simulink model "PassStFwdBkwdIsPosChk"  (R2018b)
settings: Solver=FixedStepDiscrete  StartTime=0.0  StopTime=10.0  RelTol=1e-3
undefined symbols (not defined in the file or in its folder): KeSMSuFirstRwStFwdBkwdPosDelta_Val, KeSMSuFirstRwStFwdBkwdPosTolr_Val
settings Model: Creator=sn2xws  LastModifiedBy=sn2xws
settings Model: ModifiedHistory=|
  | 2024.7.5 V3.0.0 557模式流程V1.9
  | 2024.8.14 V3.0.1 NotMovFlg从库函数中移出
settings DataIOCC: SaveFormat=StructureWithTime
settings OptimizationCC: DefaultParameterBehavior=Inlined  EnhancedBackFolding=on  PassReuseOutputArgsAs=Individual arguments  ZeroExternalMemoryAtStartup=off  ZeroInternalMemoryAtStartup=off  OptimizeBlockOrder=speed  DifferentSizesBufferReuse=on  OptimizationCustomize=off
settings DebuggingCC: ParameterTunabilityLossMsg=error
settings SFSimCC: MATLABDynamicMemAlloc=off
settings RTWCC: SystemTargetFile=autosar.tlc  GenCodeOnly=on  TemplateMakefile=ert_default_tmf  Description=AUTOSAR  GenerateReport=on  IncludeHyperlinkInReport=on  LaunchReport=on  GenerateTraceInfo=on  GenerateTraceReport=on  GenerateTraceReportSl=on  GenerateTraceReportSf=on  GenerateTraceReportEml=on
settings CodeAppCC: ForceParamTrailComments=on  IgnoreCustomStorageClasses=off  OperatorAnnotations=on  SimulinkDataObjDesc=on  SFDataObjDesc=on  InsertBlockDesc=on
settings STFCustomTargetCC: TargetLangStandard=C99 (ISO)  MultiwordLength=256  ParMdlRefBuildCompliant=on  CompOptLevelCompliant=on  IncludeMdlTerminateFcn=off  CombineOutputUpdateFcns=on  SuppressErrorStatus=on  ERTCustomFileBanners=on  SupportNonFinite=off  SupportComplex=off  SupportContinuousTime=off  SupportNonInlinedSFcns=off  RemoveResetFunc=on  MATLABClassNameForMDSCustomization=Simulink.SoftwareTarget.ERTCustomization  AutosarCompliant=on  UseToolchainInfoCompliant=on  LookupTableObjectStructAxisOrder=2,1,3,4,...  LUTObjectStructOrderEvenSpacing=Size,Table,Breakpoints  SystemTargetFile=autosar.tlc
settings ERTTargetCC: TargetLangStandard=C99 (ISO)  ConcurrentExecutionCompliant=off  IncludeMdlTerminateFcn=off  SuppressErrorStatus=on  SupportNonFinite=off  SupportComplex=off  ModelStepFunctionPrototypeControlCompliant=off  CPPClassGenCompliant=off  AutosarCompliant=on  LookupTableObjectStructAxisOrder=2,1,3,4,...  LUTObjectStructOrderEvenSpacing=Size,Table,Breakpoints  InlinedParameterPlacement=NonHierarchical  ERTCustomFileTemplate=example_file_process.tlc  ERTFilePackagingFormat=Compact

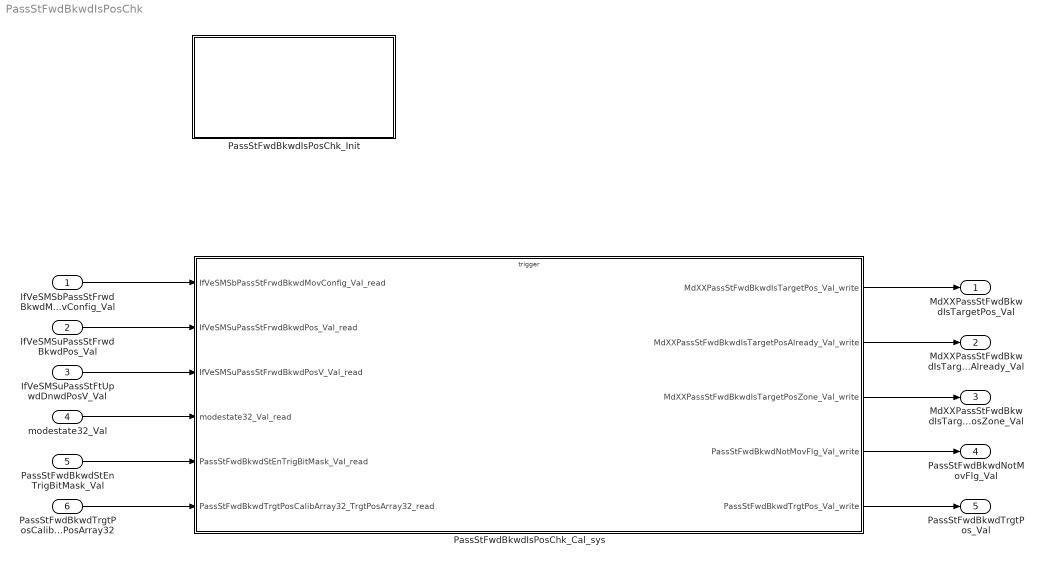
== system PassStFwdBkwdIsPosChk ==
  IfVeSMSbPassStFrwdBkwdMovConfig_Val : Inport  OutDataTypeStr=boolean  PortDimensions=1
  IfVeSMSuPassStFrwdBkwdPos_Val : Inport  Port=2  OutDataTypeStr=uint16  PortDimensions=1
  IfVeSMSuPassStFtUpwdDnwdPosV_Val : Inport  Port=3  OutDataTypeStr=boolean  PortDimensions=1
  modestate32_Val : Inport  Port=4  OutDataTypeStr=uint32  PortDimensions=1
  PassStFwdBkwdStEnTrigBitMask_Val : Inport  Port=5  OutDataTypeStr=uint32  PortDimensions=1
  PassStFwdBkwdTrgtPosCalibArray32_TrgtPosArray32 : Inport  Description=|  Port=6  OutDataTypeStr=uint16  PortDimensions=96
      | 0:Pos
      | 1:Max
      | 2:Min
  PassStFwdBkwdIsPosChk_Cal_sys : Subsystem
  PassStFwdBkwdIsPosChk_Init : Subsystem
  MdXXPassStFwdBkwdIsTargetPos_Val : Outport  OutDataTypeStr=uint32  PortDimensions=1
  MdXXPassStFwdBkwdIsTargetPosAlready_Val : Outport  Port=2  OutDataTypeStr=uint32  PortDimensions=1
  MdXXPassStFwdBkwdIsTargetPosZone_Val : Outport  Port=3  OutDataTypeStr=uint32  PortDimensions=1
  PassStFwdBkwdNotMovFlg_Val : Outport  Port=4  OutDataTypeStr=boolean  PortDimensions=1
  PassStFwdBkwdTrgtPos_Val : Outport  Port=5  OutDataTypeStr=uint16  PortDimensions=1
  wires:
  IfVeSMSbPassStFrwdBkwdMovConfig_Val/1 -> PassStFwdBkwdIsPosChk_Cal_sys/1(IfVeSMSbPassStFrwdBkwdMovConfig_Val_read)
  IfVeSMSuPassStFrwdBkwdPos_Val/1 -> PassStFwdBkwdIsPosChk_Cal_sys/2(IfVeSMSuPassStFrwdBkwdPos_Val_read)
  IfVeSMSuPassStFtUpwdDnwdPosV_Val/1 -> PassStFwdBkwdIsPosChk_Cal_sys/3(IfVeSMSuPassStFrwdBkwdPosV_Val_read)
  modestate32_Val/1 -> PassStFwdBkwdIsPosChk_Cal_sys/4(modestate32_Val_read)
  PassStFwdBkwdStEnTrigBitMask_Val/1 -> PassStFwdBkwdIsPosChk_Cal_sys/5(PassStFwdBkwdStEnTrigBitMask_Val_read)
  PassStFwdBkwdTrgtPosCalibArray32_TrgtPosArray32/1 -> PassStFwdBkwdIsPosChk_Cal_sys/6(PassStFwdBkwdTrgtPosCalibArray32_TrgtPosArray32_read)
  PassStFwdBkwdIsPosChk_Cal_sys/1(MdXXPassStFwdBkwdIsTargetPos_Val_write) -> MdXXPassStFwdBkwdIsTargetPos_Val/1
  PassStFwdBkwdIsPosChk_Cal_sys/2(MdXXPassStFwdBkwdIsTargetPosAlready_Val_write) -> MdXXPassStFwdBkwdIsTargetPosAlready_Val/1
  PassStFwdBkwdIsPosChk_Cal_sys/3(MdXXPassStFwdBkwdIsTargetPosZone_Val_write) -> MdXXPassStFwdBkwdIsTargetPosZone_Val/1
  PassStFwdBkwdIsPosChk_Cal_sys/4(PassStFwdBkwdNotMovFlg_Val_write) -> PassStFwdBkwdNotMovFlg_Val/1
  PassStFwdBkwdIsPosChk_Cal_sys/5(PassStFwdBkwdTrgtPos_Val_write) -> PassStFwdBkwdTrgtPos_Val/1

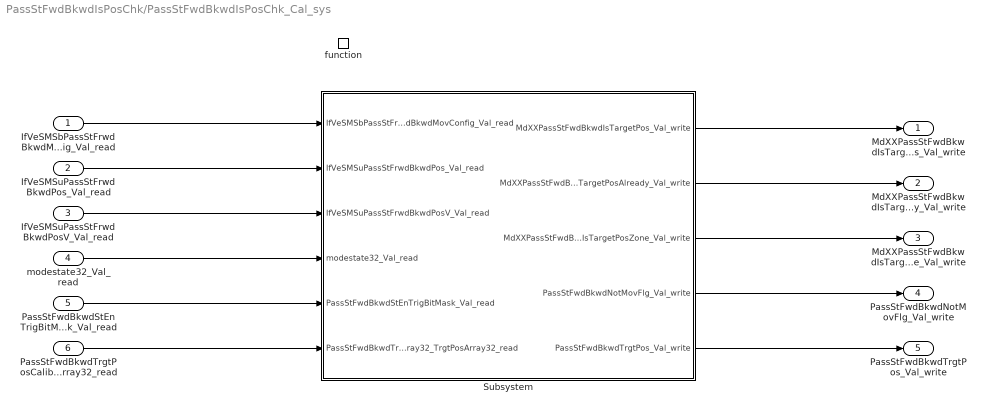
== system PassStFwdBkwdIsPosChk/PassStFwdBkwdIsPosChk_Cal_sys ==
  IfVeSMSbPassStFrwdBkwdMovConfig_Val_read : Inport
  IfVeSMSuPassStFrwdBkwdPos_Val_read : Inport  Port=2
  IfVeSMSuPassStFrwdBkwdPosV_Val_read : Inport  Port=3
  modestate32_Val_read : Inport  Port=4
  PassStFwdBkwdStEnTrigBitMask_Val_read : Inport  Port=5
  PassStFwdBkwdTrgtPosCalibArray32_TrgtPosArray32_read : Inport  Port=6
  function : TriggerPort  TriggerType=function-call  IsSimulinkFunction=on  FunctionName=PassStFwdBkwdIsPosChk_Cal  VariantControl=(inherit)
  Subsystem : Subsystem
  MdXXPassStFwdBkwdIsTargetPos_Val_write : Outport
      settings: EnsureOutportIsVirtual=on
  MdXXPassStFwdBkwdIsTargetPosAlready_Val_write : Outport  Port=2
      settings: EnsureOutportIsVirtual=on
  MdXXPassStFwdBkwdIsTargetPosZone_Val_write : Outport  Port=3
      settings: EnsureOutportIsVirtual=on
  PassStFwdBkwdNotMovFlg_Val_write : Outport  Port=4
      settings: EnsureOutportIsVirtual=on
  PassStFwdBkwdTrgtPos_Val_write : Outport  Port=5
      settings: EnsureOutportIsVirtual=on
  wires:
  IfVeSMSbPassStFrwdBkwdMovConfig_Val_read/1 -> Subsystem/1(IfVeSMSbPassStFrwdBkwdMovConfig_Val_read)
  IfVeSMSuPassStFrwdBkwdPos_Val_read/1 -> Subsystem/2(IfVeSMSuPassStFrwdBkwdPos_Val_read)
  IfVeSMSuPassStFrwdBkwdPosV_Val_read/1 -> Subsystem/3(IfVeSMSuPassStFrwdBkwdPosV_Val_read)
  modestate32_Val_read/1 -> Subsystem/4(modestate32_Val_read)
  PassStFwdBkwdStEnTrigBitMask_Val_read/1 -> Subsystem/5(PassStFwdBkwdStEnTrigBitMask_Val_read)
  PassStFwdBkwdTrgtPosCalibArray32_TrgtPosArray32_read/1 -> Subsystem/6(PassStFwdBkwdTrgtPosCalibArray32_TrgtPosArray32_read)
  Subsystem/1(MdXXPassStFwdBkwdIsTargetPos_Val_write) -> MdXXPassStFwdBkwdIsTargetPos_Val_write/1
  Subsystem/2(MdXXPassStFwdBkwdIsTargetPosAlready_Val_write) -> MdXXPassStFwdBkwdIsTargetPosAlready_Val_write/1
  Subsystem/3(MdXXPassStFwdBkwdIsTargetPosZone_Val_write) -> MdXXPassStFwdBkwdIsTargetPosZone_Val_write/1
  Subsystem/4(PassStFwdBkwdNotMovFlg_Val_write) -> PassStFwdBkwdNotMovFlg_Val_write/1
  Subsystem/5(PassStFwdBkwdTrgtPos_Val_write) -> PassStFwdBkwdTrgtPos_Val_write/1

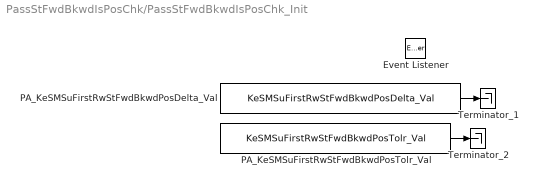
== system PassStFwdBkwdIsPosChk/PassStFwdBkwdIsPosChk_Init ==
  Event Listener : EventListener  EventName=reset
  PA_KeSMSuFirstRwStFwdBkwdPosDelta_Val : Constant  Value=KeSMSuFirstRwStFwdBkwdPosDelta_Val
  PA_KeSMSuFirstRwStFwdBkwdPosTolr_Val : Constant  Value=KeSMSuFirstRwStFwdBkwdPosTolr_Val
  Terminator_1 : Terminator
  Terminator_2 : Terminator
  wires:
  PA_KeSMSuFirstRwStFwdBkwdPosDelta_Val/1 -> Terminator_1/1
  PA_KeSMSuFirstRwStFwdBkwdPosTolr_Val/1 -> Terminator_2/1

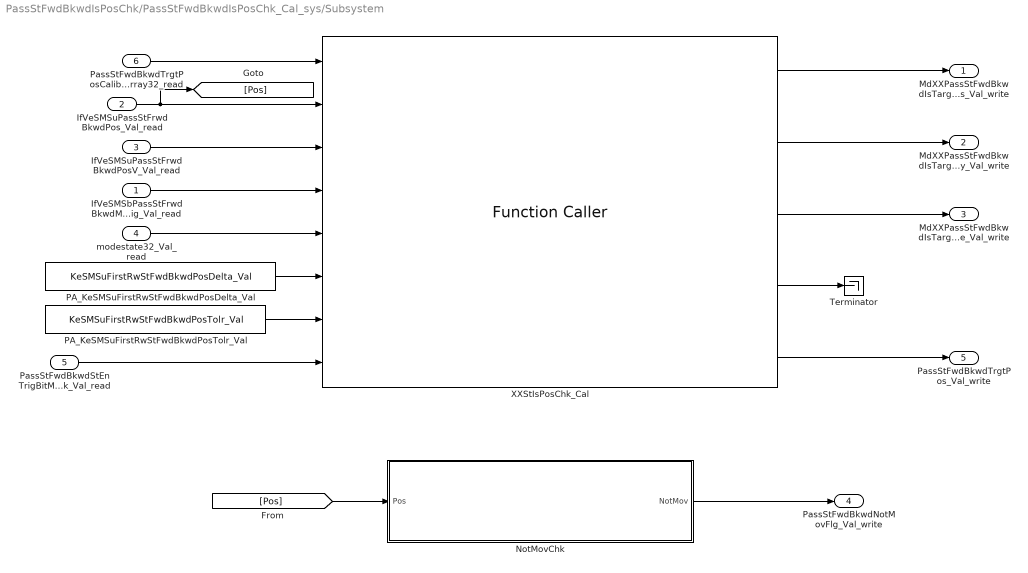
== system PassStFwdBkwdIsPosChk/PassStFwdBkwdIsPosChk_Cal_sys/Subsystem ==
  IfVeSMSbPassStFrwdBkwdMovConfig_Val_read : Inport
  IfVeSMSuPassStFrwdBkwdPos_Val_read : Inport  Port=2
  IfVeSMSuPassStFrwdBkwdPosV_Val_read : Inport  Port=3
  modestate32_Val_read : Inport  Port=4
  PassStFwdBkwdStEnTrigBitMask_Val_read : Inport  Port=5
  PassStFwdBkwdTrgtPosCalibArray32_TrgtPosArray32_read : Inport  Port=6
  NotMovChk : Subsystem
  PA_KeSMSuFirstRwStFwdBkwdPosDelta_Val : Constant  Value=KeSMSuFirstRwStFwdBkwdPosDelta_Val
  PA_KeSMSuFirstRwStFwdBkwdPosTolr_Val : Constant  Value=KeSMSuFirstRwStFwdBkwdPosTolr_Val
  Terminator : Terminator
  XXStIsPosChk_Cal : FunctionCaller  FunctionPrototype=[IsPos,IsPosAlready,IsPosZone,NotMovFlg,StTrgtPos] = XXStIsPosChk_Cal(MdCalibArray32,Pos,PosV,MovConfig,modestate32,PosDelta,PosTolr,StBitMask)  InputArgumentSpecifications=uint16([1;1;1;1;1;1;1;1;1;1;1;1;1;1;1;1;1;1;1;1;1;1;1;1;1;1;1;1;1;1;1;1;1;1;1;1;1;1;1;1;1;1;1;1;1;1;1;1;1;1;1;1;1;1;1;1;1;1;1;1;1;1;1;1;1;1;1;1;1;1;1;1;1;1;1;1;1;1;1;1;1;1;1;1;1;1;1;1;1;1;1;1;1;1;1;1]), uint16(1), boolean(true), boolean(true), uint32(1), uint16(1), uint16(1), uint32(1)  OutputArgumentSpecifications=uint32(1), uint32(1), uint32(1), boolean(true), uint16(1)
  MdXXPassStFwdBkwdIsTargetPos_Val_write : Outport
      settings: EnsureOutportIsVirtual=on
  MdXXPassStFwdBkwdIsTargetPosAlready_Val_write : Outport  Port=2
      settings: EnsureOutportIsVirtual=on
  MdXXPassStFwdBkwdIsTargetPosZone_Val_write : Outport  Port=3
      settings: EnsureOutportIsVirtual=on
  PassStFwdBkwdNotMovFlg_Val_write : Outport  Port=4
      settings: EnsureOutportIsVirtual=on
  PassStFwdBkwdTrgtPos_Val_write : Outport  Port=5
      settings: EnsureOutportIsVirtual=on
  wires:
  IfVeSMSuPassStFrwdBkwdPosV_Val_read/1 -> XXStIsPosChk_Cal/3
  PassStFwdBkwdStEnTrigBitMask_Val_read/1 -> XXStIsPosChk_Cal/8
  IfVeSMSuPassStFrwdBkwdPos_Val_read/1 -> [Pos], XXStIsPosChk_Cal/2
  PA_KeSMSuFirstRwStFwdBkwdPosDelta_Val/1 -> XXStIsPosChk_Cal/6
  modestate32_Val_read/1 -> XXStIsPosChk_Cal/5
  PassStFwdBkwdTrgtPosCalibArray32_TrgtPosArray32_read/1 -> XXStIsPosChk_Cal/1
  PA_KeSMSuFirstRwStFwdBkwdPosTolr_Val/1 -> XXStIsPosChk_Cal/7
  IfVeSMSbPassStFrwdBkwdMovConfig_Val_read/1 -> XXStIsPosChk_Cal/4
  XXStIsPosChk_Cal/1 -> MdXXPassStFwdBkwdIsTargetPos_Val_write/1
  XXStIsPosChk_Cal/2 -> MdXXPassStFwdBkwdIsTargetPosAlready_Val_write/1
  XXStIsPosChk_Cal/3 -> MdXXPassStFwdBkwdIsTargetPosZone_Val_write/1
  XXStIsPosChk_Cal/5 -> PassStFwdBkwdTrgtPos_Val_write/1
  [Pos] -> NotMovChk/1(Pos)
  NotMovChk/1(NotMov) -> PassStFwdBkwdNotMovFlg_Val_write/1
  XXStIsPosChk_Cal/4 -> Terminator/1

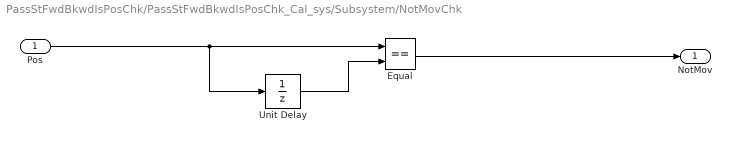
== system PassStFwdBkwdIsPosChk/PassStFwdBkwdIsPosChk_Cal_sys/Subsystem/NotMovChk ==
  Pos : Inport
  Equal : RelationalOperator  Operator===  OutDataTypeStr=boolean  RndMeth=Simplest
  Unit Delay : UnitDelay  SampleTime=-1
  NotMov : Outport
  wires:
  Unit Delay/1 -> Equal/2
  Pos/1 -> Unit Delay/1, Equal/1
  Equal/1 -> NotMov/1
